simulink model "MSX60_10_RL"  (Simulink 7.9)
settings: Solver=ode14x  StartTime=0.0  StopTime=250  FixedStep=0.05  RelTol=1e-4
values from neighbouring files (symbols this model uses):
  n = 1.3    [MSX60DS.m]    (also in MSX60_10_RL.m; MSX60_10_by2_with_PandO.m; MSX60_10_by2_with_PandO_PS.m; MSX60_10_by2_with_PandO_US (1).m)
  Ns = 1    [MSX60DS.m]    (also in MSX60_10_RL.m; MSX60_10_by2_with_PandO.m; MSX60_10_by2_with_PandO_PS.m; MSX60_10_by2_with_PandO_US (1).m)
  Rs = 0.58    [MSX60DS.m]    (also in MSX60_10_RL.m; MSX60_10_by2_with_PandO.m; MSX60_10_by2_with_PandO_PS.m; MSX60_10_by2_with_PandO_US (1).m)
  Voc = Voc(1)    [MSX60DS.m]    (also in MSX60_10_RL.m = 21.1; MSX60_10_by2_with_PandO.m = 21.1; MSX60_10_by2_with_PandO_PS.m = 21.1; MSX60_10_by2_with_PandO_US (1).m = 21.1)
libraries: fl_lib x15, elec_lib x10, nesl_utility x4, simulink x1
settings Model: Creator=pc1  LastModifiedBy=91940
settings SolverCC: SolverJacobianMethodControl=SparsePerturbation
settings DataIOCC: SaveState=on

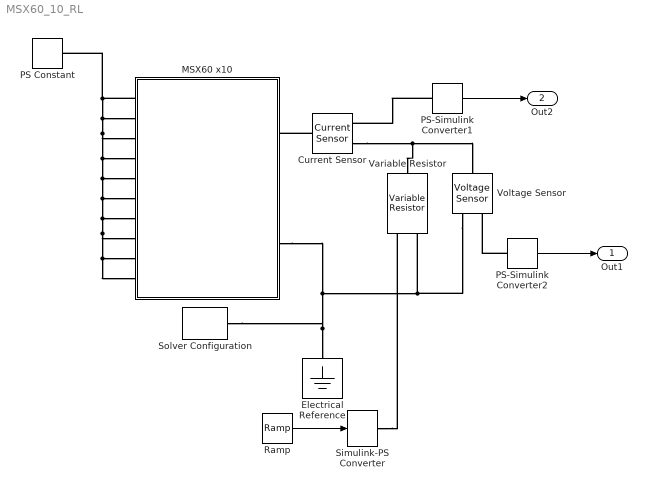
== system MSX60_10_RL ==
  Current Sensor : fl_lib/Electrical/Electrical Sensors/Current Sensor  i1_Log=off  v1_Log=off  LocalVarNames=|i1|v1  LocalVarDescs=|i1|v1  LocalVarLogging=[0 0]
  Electrical Reference : fl_lib/Electrical/Electrical Elements/Electrical Reference  i_Log=off  LocalVarNames=|i  LocalVarDescs=|i  LocalVarLogging=0
  MSX60 x10 : Subsystem
  PS Constant : fl_lib/Physical Signals/Sources/PS Constant  constant=G  LocalVarLogging=[]
  PS-Simulink Converter1 : nesl_utility/PS-Simulink Converter  PhysicalDomain=network_engine_domain  LeftPortType=input  RightPortType=output  SubClassName=ps_output  Unit=1  AffineConversion=off
  PS-Simulink Converter2 : nesl_utility/PS-Simulink Converter  PhysicalDomain=network_engine_domain  LeftPortType=input  RightPortType=output  SubClassName=ps_output  Unit=1  AffineConversion=off
  Ramp : simulink/Sources/Ramp  slope=0.22  start=0  X0=0
  Simulink-PS Converter : nesl_utility/Simulink-PS Converter  PhysicalDomain=network_engine_domain  LeftPortType=input  RightPortType=output  SubClassName=ps_input  Unit=1  AffineConversion=off  InputFilterTimeConstant=.001  UdotUserProvided=[]  SimscapeFilterOrder=1  InputFiltering=off
  Solver Configuration : nesl_utility/Solver Configuration  PhysicalDomain=network_engine_domain  LeftPortType=input  RightPortType=generic  SubClassName=solver  UseCustomDae=off  DoDC=on  ResidualTolerance=1e-9  UseLocalSolver=off  LocalSolverChoice=NE_BACKWARD_EULER_ADVANCER  LocalSolverSampleTime=.001  DoFixedCost=off  MaxNonlinIter=3  MaxModeIter=2  LinearAlgebra=Sparse  Accelerate=off  Profile=off  UseLocalSampling=off  DelaysMemoryBudget=1024
  Variable Resistor : fl_lib/Electrical/Electrical Elements/Variable Resistor  Rmin=0 Ohm  i_Log=off  v_Log=off  LocalVarNames=|i|v  LocalVarDescs=|i|v  LocalVarLogging=[0 0]
  Voltage Sensor : fl_lib/Electrical/Electrical Sensors/Voltage Sensor  i1_Log=off  v1_Log=off  LocalVarNames=|i1|v1  LocalVarDescs=|i1|v1  LocalVarLogging=[0 0]
  Out1 : Outport
  Out2 : Outport  Port=2
  wires:
  PS-Simulink Converter1/1 -> Out2/1
  Ramp/1 -> Simulink-PS Converter/1
  PS-Simulink Converter2/1 -> Out1/1
  connections:
  Current Sensor/RConn2 -- Variable Resistor/RConn1 -- Voltage Sensor/LConn1
  MSX60 x10/LConn1 -- PS Constant/RConn1 -- MSX60 x10/LConn2 -- MSX60 x10/LConn3 -- MSX60 x10/LConn4 -- MSX60 x10/LConn5 -- MSX60 x10/LConn6 -- MSX60 x10/LConn7 -- MSX60 x10/LConn8 -- MSX60 x10/LConn9 -- MSX60 x10/LConn10
  Current Sensor/LConn1 -- MSX60 x10/RConn1
  MSX60 x10/RConn2 -- Electrical Reference/LConn1 -- Solver Configuration/RConn1 -- Variable Resistor/LConn2 -- Voltage Sensor/RConn2
  Simulink-PS Converter/RConn1 -- Variable Resistor/LConn1
  PS-Simulink Converter2/LConn1 -- Voltage Sensor/RConn1
  PS-Simulink Converter1/LConn1 -- Current Sensor/RConn1

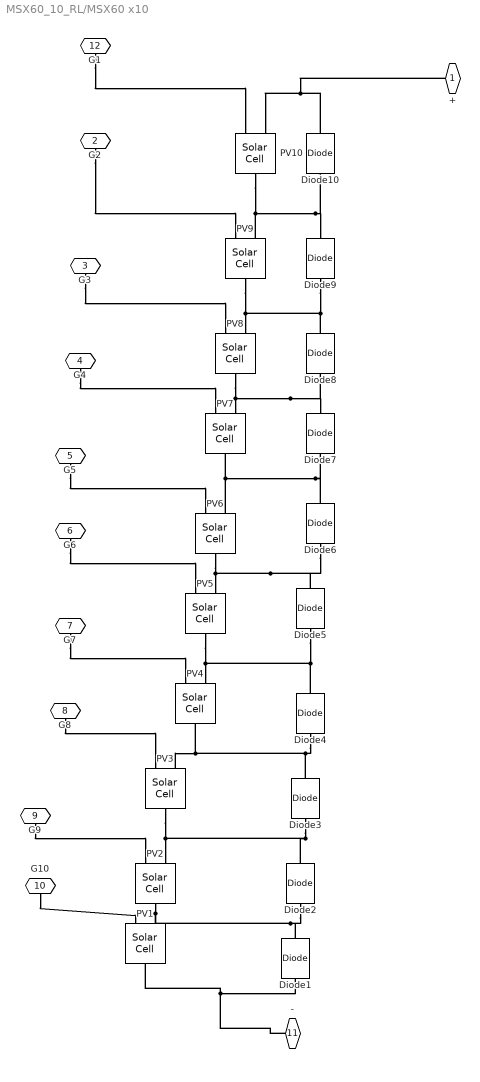
== system MSX60_10_RL/MSX60 x10 ==
  Diode{1..10} (10 alike) : fl_lib/Electrical/Electrical Elements/Diode  Vf=0.6 V  Ron=0.3 Ohm  Goff=1e-8 1/Ohm  i_Log=off  v_Log=off  LocalVarNames=|i|v  LocalVarDescs=|i|v  LocalVarLogging=[0 0]
  PV{1..10} (10 alike) : elec_lib/Sources/Solar Cell  prm=1  Isc=Isc A  Voc=Voc*Ns V  Is=1e-6 A  Is2=0 A  Iph=3.8 A  Ir0=Gstc W/m^2  ec=n*Voc*Ns  N2=0  Rs=Rs*Ns Ohm  Rp=Inf Ohm  TIPH1=0 1/K  EG=1.11 eV  TXIS1=3  TXIS2=3  TRS1=0  TRP1=0  Tmeas=25 C  TFIXED=25 C  LocalVarLogging=[]  thermal_mass=100 J/K  initial_temperature=25 C
  + : PMIOPort  Port=1  Side=Right
  G2 : PMIOPort  Port=2  Side=Left
  G3 : PMIOPort  Port=3  Side=Left
  G4 : PMIOPort  Port=4  Side=Left
  G5 : PMIOPort  Port=5  Side=Left
  G6 : PMIOPort  Port=6  Side=Left
  G7 : PMIOPort  Port=7  Side=Left
  G8 : PMIOPort  Port=8  Side=Left
  G9 : PMIOPort  Port=9  Side=Left
  G10 : PMIOPort  Port=10  Side=Left
  - : PMIOPort  Port=11  Side=Right
  G1 : PMIOPort  Port=12  Side=Left
  connections:
  Diode4/LConn1 -- PV3/LConn2 -- PV4/RConn1 -- Diode3/RConn1
  Diode5/LConn1 -- PV5/RConn1 -- PV4/LConn2 -- Diode4/RConn1
  Diode6/LConn1 -- PV6/RConn1 -- PV5/LConn2 -- Diode5/RConn1
  PV8/RConn1 -- PV7/LConn2 -- Diode7/RConn1 -- Diode8/LConn1
  Diode9/LConn1 -- PV8/LConn2 -- PV9/RConn1 -- Diode8/RConn1
  G10/RConn1 -- PV1/LConn1
  -/RConn1 -- PV1/RConn1 -- Diode1/LConn1
  G9/RConn1 -- PV2/LConn1
  Diode2/LConn1 -- PV2/RConn1 -- PV1/LConn2 -- Diode1/RConn1
  Diode3/LConn1 -- PV2/LConn2 -- PV3/RConn1 -- Diode2/RConn1
  G8/RConn1 -- PV3/LConn1
  PV6/LConn2 -- PV7/RConn1 -- Diode7/LConn1 -- Diode6/RConn1
  PV9/LConn2 -- PV10/RConn1 -- Diode9/RConn1 -- Diode10/LConn1
  Diode10/RConn1 -- PV10/LConn2 -- +/RConn1
  G7/RConn1 -- PV4/LConn1
  G6/RConn1 -- PV5/LConn1
  G5/RConn1 -- PV6/LConn1
  G4/RConn1 -- PV7/LConn1
  G3/RConn1 -- PV8/LConn1
  G2/RConn1 -- PV9/LConn1
  G1/RConn1 -- PV10/LConn1
